simulink model "Robot3GDL"  (R2022a)
settings: Solver=VariableStepAuto  StartTime=0.0  StopTime=Tfinal  RelTol=1e-3
undefined symbols (not defined in the file or in its folder): Cilindric_mgd, MGI, Tem
settings Model: Creator=Shadow  LastModifiedBy=Shadow
settings DebuggingCC: UnconnectedInputMsg=warning  UnconnectedOutputMsg=warning  UnconnectedLineMsg=warning
settings RTWCC: DLArmComputeVersion=19.05

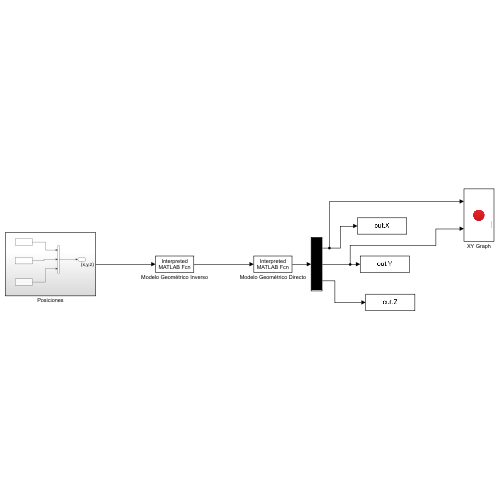
[thumbnail: Simulink's stored preview of the top-level diagram]
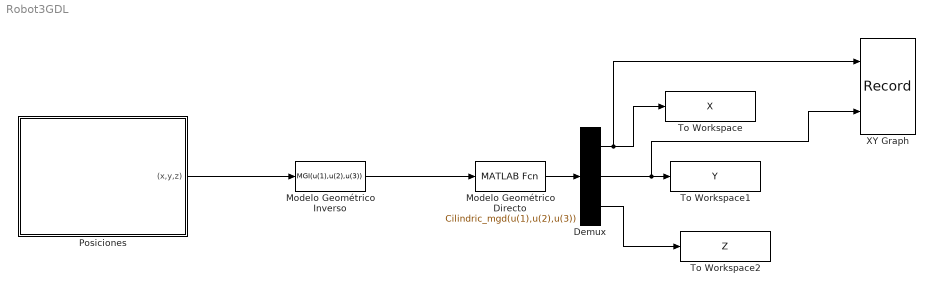
== system Robot3GDL ==
  Demux : Demux  Outputs=3
  Modelo Geométrico Directo : MATLABFcn  MATLABFcn=Cilindric_mgd(u(1),u(2),u(3))  OutputDimensions=3
  Modelo Geométrico Inverso : MATLABFcn  MATLABFcn=MGI(u(1),u(2),u(3))  OutputDimensions=3
  Posiciones : Subsystem
  To Workspace : ToWorkspace  VariableName=X
  To Workspace1 : ToWorkspace  VariableName=Y
  To Workspace2 : ToWorkspace  VariableName=Z
  XY Graph : Record  FileSettingsInternal="{\"entries\":[{\"content\":{\"excelSettings\":{\"content\":{},\"type\":\"Streamout.ExcelSettings\"}},\"type\":\"Streamout.FileSettingStorage\",\"uuid\":\"146d7f99-7208-4f55-a6e8-6304b15e4bd9\"}],\"packageUris\":[\"http://schema.mathworks.com/mf0/streamout_blocks/R2020a\"],\"version\":\"1.0\"}"  Layout=[1 1]  SignalsInternal="{\"entries\":[{\"content\":{\"signals\":[{\"content\":{\"blockPath\":[\"Robot3GDL/XY Graph\"],\"channel\":[],\"dimensions\":[1],\"domain\":\"Robot3GDL/XY Graph\",\"lineColor\":\"#a2142f\",\"plots\":[1],\"port\":1,\"sid\":[\"\"],\"signalID\":227,\"signalName\":\"Demux:1\"},\"type\":\"RecordBlkView.Signal\",\"uuid\":\"c8ec3325-1740-43f1-8bca-6232c06e123b\"},{\"content\":{\"blockPath\":[\"Robot3GDL/XY Graph\"],\"channel\":[],\"dimensions\":[1],\"domain\":\"Robot3GDL/XY Graph\",\"lineColor\":\"#139fff\",\"plots\":[1],\"port\":2,\"sid\":[\"\"],\"signalID\":231,\"signalName\":\"Demux:2\"},\"type\":\"RecordBlkView.Signal\",\"uuid\":\"0000bffe-2f5b-4cf6-ba1f-35aef20620b9\"}]},\"type\":\"RecordBlkView.InputSignals\",\"uuid\":\"c2abdf48-26d1-4f92-b126-64282879f8ff\"}],\"packageUris\":[\"http://schema.mathworks.com/mf0/streamout_blocks/R2020a\"],\"version\":\"1.0\"}"  VisualizationBindings="{\"xyplotplugin\":{\"info\":[{\"series\":[{\"bindingParametersList\":[{\"parameter\":\"X-Axis\",\"signalID\":227,\"signalName\":\"Demux:1\"},{\"parameter\":\"Y-Axis\",\"signalID\":231,\"signalName\":\"Demux:2\"}],\"seriesID\":387}],\"subplotID\":1}]}}"  CompatibilityTag=XY
  wires:
  Demux/2 -> XY Graph/2, To Workspace1/1
  Demux/3 -> To Workspace2/1
  Modelo Geométrico Directo/1 -> Demux/1
  Modelo Geométrico Inverso/1 -> Modelo Geométrico Directo/1
  Posiciones/1((x,y,z)) -> Modelo Geométrico Inverso/1
  Demux/1 -> To Workspace/1, XY Graph/1

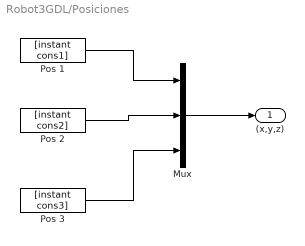
== system Robot3GDL/Posiciones ==
  Mux : Mux  Inputs=3
  Pos 1 : FromWorkspace  VariableName=[instant cons1]  SampleTime=Tem  ZeroCross=off
  Pos 2 : FromWorkspace  VariableName=[instant cons2]  SampleTime=Tem  ZeroCross=off
  Pos 3 : FromWorkspace  VariableName=[instant cons3]  SampleTime=Tem  ZeroCross=off
  (x,y,z) : Outport
  wires:
  Pos 3/1 -> Mux/3
  Pos 1/1 -> Mux/1
  Pos 2/1 -> Mux/2
  Mux/1 -> (x,y,z)/1
